simulink model "EST"  (R2025a)
settings: Solver=FixedStepAuto  StartTime=0.0  StopTime=stopt  FixedStep=deltat  MaxStep=0.05  RelTol=1e-3
InitFcn:
  | clear all;
  | close all;
  | clc;
  | 
  | % add the data and script directories
  | addpath('data','scripts');
  | 
  | % load the constants (units)
  | constants;
  | 
  | % load the simulation parameters
  | preprocessing;
StopFcn:
  | postprocessing;
values from neighbouring files (symbols this model uses):
  aDemandTransport = 0.01    [preprocessing.m]
  aInjection = 0.2    [preprocessing.m]
  aSupplyTransport = 0.01    [preprocessing.m]
  bStorage = (1/(ro*V*c*Rtb))/unit("s")    [preprocessing.m]
  EStorageInitial = 0.0*unit("MWh")    [preprocessing.m]
  EStorageMax = 107.*unit("MWh")    [preprocessing.m]
  EStorageMin = 0.1*unit("MWh")    [preprocessing.m]
settings Model: Creator=joche  LastModifiedBy=20253517
settings DataIOCC: SaveFormat=Array  SaveOutput=off  ReturnWorkspaceOutputs=off
settings OptimizationCC: ReuseModelBlockBuffer=off
settings ModelReferenceCC: EnableRefExpFcnMdlSchedulingChecks=on
settings RTWCC: GPUComputeCapability=3.5

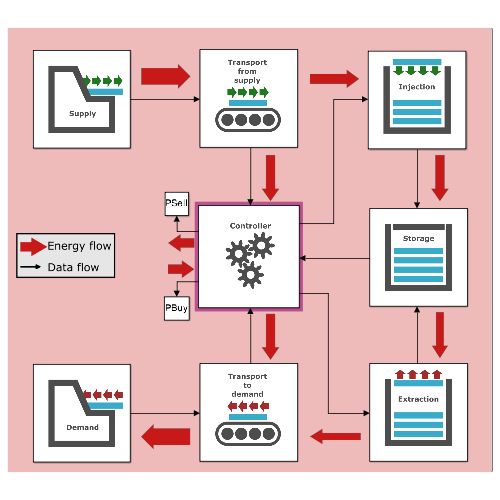
[thumbnail: Simulink's stored preview of the top-level diagram]
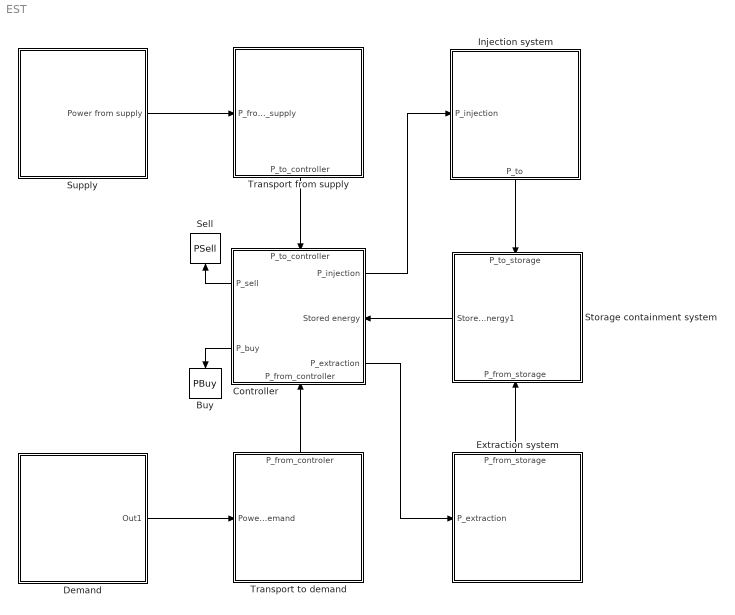
== system EST ==
  Buy : ToWorkspace  VariableName=PBuy  SampleTime=-1
  Controller : Subsystem
      settings: PortSchema="{\"entries\":[{\"content\":{\"sides\":[{\"content\":{\"connectorIds\":[\"Out3\",\"Out4\"]},\"type\":\"ConnectorPlacement.EquallySpacedRectSide\",\"uuid\":\"4daf33ce-c96a-4783-b5c4-228eed953e01\"},{\"content\":{\"connectorIds\":[\"Out1\",\"In3\",\"Out2\"],\"side\":\"RIGHT\"},\"type\":\"ConnectorPlacement.EquallySpacedRectSide\",\"uuid\":\"e9942e50-8467-4af8-b79b-80636cbc76e5\"},{\"content\":{\"connectorIds\":[\"In1\"],\"side\":\"TOP\"},\"type\":\"ConnectorPlacement.EquallySpacedRectSide\",\"uuid\":\"f315e931-d69b-4751-b712-f89c6c81baeb\"},{\"content\":{\"connectorIds\":[\"In2\"],\"side\":\"BOTTOM\"},\"type\":\"ConnectorPlacement.EquallySpacedRectSide\",\"uuid\":\"44715ee6-5cd5-4669-bcb9-5ed7c869bdb3\"}]},\"type\":\"ConnectorPlacement.EquallySpacedConnector\",\"uuid\":\"fff48899-944b-4064-b7d7-ecc12144fb48\"}],\"packageUris\":[\"http://schema.mathworks.com/mf0/Connector/R2020b\"],\"version\":\"1.0\"}"
      mask Display: image('$imagefile'); % Use "Edit Image" on toolstrip to change.
  Demand : Subsystem
      mask Display: image('$imagefile'); % Use "Edit Image" on toolstrip to change.
  Extraction system : Subsystem
      settings: PortSchema="{\"entries\":[{\"content\":{\"sides\":[{\"content\":{\"connectorIds\":[]},\"type\":\"ConnectorPlacement.EquallySpacedRectSide\",\"uuid\":\"05c5933d-55fc-4e06-853f-fc26d42905f9\"},{\"content\":{\"connectorIds\":[\"In1\"],\"side\":\"RIGHT\"},\"type\":\"ConnectorPlacement.EquallySpacedRectSide\",\"uuid\":\"327426c5-31d5-498b-a2bd-83e49353408c\"},{\"content\":{\"connectorIds\":[],\"side\":\"TOP\"},\"type\":\"ConnectorPlacement.EquallySpacedRectSide\",\"uuid\":\"55306cf3-a3de-4385-a5ae-b8600ecdd5a2\"},{\"content\":{\"connectorIds\":[\"Out1\"],\"side\":\"BOTTOM\"},\"type\":\"ConnectorPlacement.EquallySpacedRectSide\",\"uuid\":\"08fcc9c3-40d3-4ac6-b914-dfeef6039ffb\"}]},\"type\":\"ConnectorPlacement.EquallySpacedConnector\",\"uuid\":\"cb35d5ba-e8c6-462c-b7b2-fe8356d4b0a1\"}],\"packageUris\":[\"http://schema.mathworks.com/mf0/Connector/R2020b\"],\"version\":\"1.0\"}"
      mask Display: image('$imagefile'); % Use "Edit Image" on toolstrip to change.
  Injection system : Subsystem
      settings: PortSchema="{\"entries\":[{\"content\":{\"sides\":[{\"content\":{\"connectorIds\":[]},\"type\":\"ConnectorPlacement.EquallySpacedRectSide\",\"uuid\":\"05c5933d-55fc-4e06-853f-fc26d42905f9\"},{\"content\":{\"connectorIds\":[\"In1\"],\"side\":\"RIGHT\"},\"type\":\"ConnectorPlacement.EquallySpacedRectSide\",\"uuid\":\"327426c5-31d5-498b-a2bd-83e49353408c\"},{\"content\":{\"connectorIds\":[\"Out1\"],\"side\":\"TOP\"},\"type\":\"ConnectorPlacement.EquallySpacedRectSide\",\"uuid\":\"55306cf3-a3de-4385-a5ae-b8600ecdd5a2\"},{\"content\":{\"connectorIds\":[],\"side\":\"BOTTOM\"},\"type\":\"ConnectorPlacement.EquallySpacedRectSide\",\"uuid\":\"08fcc9c3-40d3-4ac6-b914-dfeef6039ffb\"}]},\"type\":\"ConnectorPlacement.EquallySpacedConnector\",\"uuid\":\"cb35d5ba-e8c6-462c-b7b2-fe8356d4b0a1\"}],\"packageUris\":[\"http://schema.mathworks.com/mf0/Connector/R2020b\"],\"version\":\"1.0\"}"
      mask Display: image('$imagefile'); % Use "Edit Image" on toolstrip to change.
  Sell : ToWorkspace  VariableName=PSell  SampleTime=-1
  Storage containment system : Subsystem
      settings: PortSchema="{\"entries\":[{\"content\":{\"sides\":[{\"content\":{\"connectorIds\":[\"Out1\"]},\"type\":\"ConnectorPlacement.EquallySpacedRectSide\",\"uuid\":\"0ba48424-33b9-4934-970f-64fe5d8b070e\"},{\"content\":{\"connectorIds\":[],\"side\":\"RIGHT\"},\"type\":\"ConnectorPlacement.EquallySpacedRectSide\",\"uuid\":\"9cde340f-8f39-4499-9a12-5e1623737660\"},{\"content\":{\"connectorIds\":[\"In1\"],\"side\":\"TOP\"},\"type\":\"ConnectorPlacement.EquallySpacedRectSide\",\"uuid\":\"2af8db04-7fd0-4902-8637-8dc00edb4598\"},{\"content\":{\"connectorIds\":[\"In2\"],\"side\":\"BOTTOM\"},\"type\":\"ConnectorPlacement.EquallySpacedRectSide\",\"uuid\":\"e21ea806-d777-41a3-a53f-556fae66854b\"}]},\"type\":\"ConnectorPlacement.EquallySpacedConnector\",\"uuid\":\"4e2ddb36-4db3-4ab4-858b-ebb8ccefeb1f\"}],\"packageUris\":[\"http://schema.mathworks.com/mf0/Connector/R2020b\"],\"version\":\"1.0\"}"
      mask Display: image('$imagefile'); % Use "Edit Image" on toolstrip to change.
  Supply : Subsystem
      mask Display: image('$imagefile'); % Use "Edit Image" on toolstrip to change.
  Transport from supply : Subsystem
      settings: PortSchema="{\"entries\":[{\"content\":{\"sides\":[{\"content\":{\"connectorIds\":[\"In1\"]},\"type\":\"ConnectorPlacement.EquallySpacedRectSide\",\"uuid\":\"31329006-3d36-4d93-9c44-7503a515d397\"},{\"content\":{\"connectorIds\":[],\"side\":\"RIGHT\"},\"type\":\"ConnectorPlacement.EquallySpacedRectSide\",\"uuid\":\"aba139c7-f9b6-4881-a56b-a4cbbedacd88\"},{\"content\":{\"connectorIds\":[],\"side\":\"TOP\"},\"type\":\"ConnectorPlacement.EquallySpacedRectSide\",\"uuid\":\"e683eb73-7a35-4160-9c39-da83856a6278\"},{\"content\":{\"connectorIds\":[\"Out1\"],\"side\":\"BOTTOM\"},\"type\":\"ConnectorPlacement.EquallySpacedRectSide\",\"uuid\":\"1170dd18-447c-437f-9043-6812c2877331\"}]},\"type\":\"ConnectorPlacement.EquallySpacedConnector\",\"uuid\":\"804af608-1d70-444f-af69-e05f19bf98f3\"}],\"packageUris\":[\"http://schema.mathworks.com/mf0/Connector/R2020b\"],\"version\":\"1.0\"}"
      mask Display: image('$imagefile'); % Use "Edit Image" on toolstrip to change.
  Transport to demand : Subsystem
      settings: PortSchema="{\"entries\":[{\"content\":{\"sides\":[{\"content\":{\"connectorIds\":[\"In1\"]},\"type\":\"ConnectorPlacement.EquallySpacedRectSide\",\"uuid\":\"31329006-3d36-4d93-9c44-7503a515d397\"},{\"content\":{\"connectorIds\":[],\"side\":\"RIGHT\"},\"type\":\"ConnectorPlacement.EquallySpacedRectSide\",\"uuid\":\"aba139c7-f9b6-4881-a56b-a4cbbedacd88\"},{\"content\":{\"connectorIds\":[\"Out1\"],\"side\":\"TOP\"},\"type\":\"ConnectorPlacement.EquallySpacedRectSide\",\"uuid\":\"e683eb73-7a35-4160-9c39-da83856a6278\"},{\"content\":{\"connectorIds\":[],\"side\":\"BOTTOM\"},\"type\":\"ConnectorPlacement.EquallySpacedRectSide\",\"uuid\":\"c378138f-7233-4483-870c-40a69b3495ee\"}]},\"type\":\"ConnectorPlacement.EquallySpacedConnector\",\"uuid\":\"804af608-1d70-444f-af69-e05f19bf98f3\"}],\"packageUris\":[\"http://schema.mathworks.com/mf0/Connector/R2020b\"],\"version\":\"1.0\"}"
      mask Display: image('$imagefile'); % Use "Edit Image" on toolstrip to change.
  wires:
  Supply/1(Power from supply) -> Transport from supply/1(P_from_supply)
  Transport from supply/1(P_to_controller) -> Controller/1(P_to_controller)
  Transport to demand/1(P_from_controler) -> Controller/2(P_from_controller)
  Demand/1(Out1) -> Transport to demand/1(Power to demand)
  Controller/3(P_sell) -> Sell/1
  Controller/2(P_extraction) -> Extraction system/1(P_extraction)
  Injection system/1(P_to) -> Storage containment system/1(P_to_storage)
  Extraction system/1(P_from_storage) -> Storage containment system/2(P_from_storage)
  Storage containment system/1(Stored energy1) -> Controller/3(Stored energy)
  Controller/1(P_injection) -> Injection system/1(P_injection)
  Controller/4(P_buy) -> Buy/1

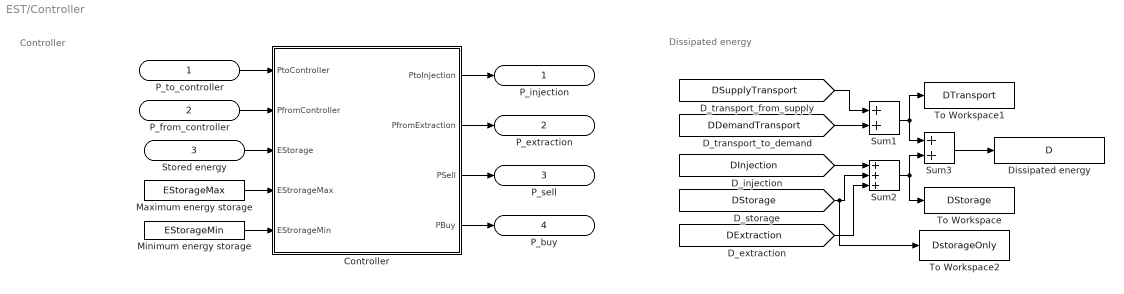
== system EST/Controller ==
  note: Dissipated energy
  note: Controller
  P_to_controller : Inport
  P_from_controller : Inport  Port=2
  Stored energy : Inport  Port=3
  Controller : MATLAB Function  TreatAsAtomicUnit=on
  Dissipated energy : ToWorkspace  VariableName=D  SampleTime=-1
  Maximum energy storage : Constant  Value=EStorageMax
  Minimum energy storage : Constant  Value=EStorageMin
  Sum1 : Sum
  Sum2 : Sum  Inputs=+++
  Sum3 : Sum
  To Workspace : ToWorkspace  VariableName=DStorage  SampleTime=-1
  To Workspace1 : ToWorkspace  VariableName=DTransport  SampleTime=-1
  To Workspace2 : ToWorkspace  VariableName=DstorageOnly  SampleTime=-1
  P_injection : Outport
  P_extraction : Outport  Port=2
  P_sell : Outport  Port=3
  P_buy : Outport  Port=4
  wires:
  P_from_controller/1 -> Controller/2(PfromController)
  Controller/2(PfromExtraction) -> P_extraction/1
  Controller/3(PSell) -> P_sell/1
  Controller/4(PBuy) -> P_buy/1
  Minimum energy storage/1 -> Controller/5(EStrorageMin)
  Maximum energy storage/1 -> Controller/4(EStrorageMax)
  P_to_controller/1 -> Controller/1(PtoController)
  Controller/1(PtoInjection) -> P_injection/1
  Stored energy/1 -> Controller/3(EStorage)
  [DDemandTransport] -> Sum1/2
  [DSupplyTransport] -> Sum1/1
  [DInjection] -> Sum2/1
  [DStorage] -> To Workspace2/1, Sum2/2
  [DExtraction] -> Sum2/3
  Sum2/1 -> To Workspace/1, Sum3/2
  Sum1/1 -> To Workspace1/1, Sum3/1
  Sum3/1 -> Dissipated energy/1

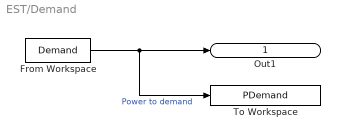
== system EST/Demand ==
  From Workspace : FromWorkspace  VariableName=Demand  OutputAfterFinalValue=Setting to zero
  To Workspace : ToWorkspace  VariableName=PDemand  SampleTime=-1
  Out1 : Outport
  wires:
  From Workspace/1 -> To Workspace/1, Out1/1  "Power to demand"

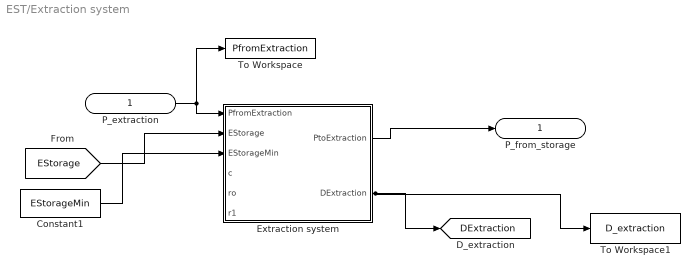
== system EST/Extraction system ==
  P_extraction : Inport
  Constant1 : Constant  Value=EStorageMin
  Extraction system : MATLAB Function  TreatAsAtomicUnit=on
  To Workspace : ToWorkspace  VariableName=PfromExtraction  SampleTime=-1
  To Workspace1 : ToWorkspace  VariableName=D_extraction  SampleTime=-1
  P_from_storage : Outport
  tag scope: DExtraction=global
  wires:
  P_extraction/1 -> To Workspace/1, Extraction system/1(PfromExtraction)
  Extraction system/1(PtoExtraction) -> P_from_storage/1
  [EStorage] -> Extraction system/2(EStorage)
  Constant1/1 -> Extraction system/3(EStorageMin)
  Extraction system/2(DExtraction) -> To Workspace1/1, [DExtraction]

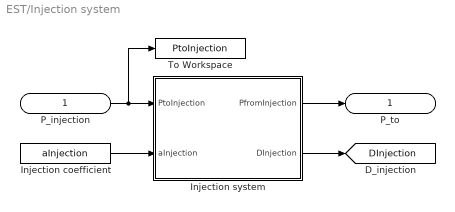
== system EST/Injection system ==
  P_injection : Inport
  Injection coefficient : Constant  Value=aInjection
  Injection system : MATLAB Function  TreatAsAtomicUnit=on
  To Workspace : ToWorkspace  VariableName=PtoInjection  SampleTime=-1
  P_to : Outport
  tag scope: DInjection=global
  wires:
  P_injection/1 -> To Workspace/1, Injection system/1(PtoInjection)
  Injection system/1(PfromInjection) -> P_to/1
  Injection coefficient/1 -> Injection system/2(aInjection)
  Injection system/2(DInjection) -> [DInjection]

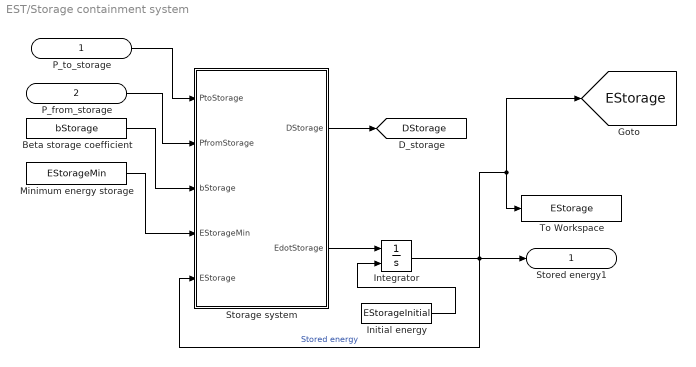
== system EST/Storage containment system ==
  P_to_storage : Inport
  P_from_storage : Inport  Port=2
  Beta storage coefficient : Constant  Value=bStorage
  Initial energy : Constant  Value=EStorageInitial
  Integrator : Integrator  InitialConditionSource=external
  Minimum energy storage : Constant  Value=EStorageMin
  Storage system : MATLAB Function  TreatAsAtomicUnit=on
  To Workspace : ToWorkspace  VariableName=EStorage  SampleTime=-1
  Stored energy1 : Outport
  tag scope: DStorage=global, EStorage=global
  wires:
  P_from_storage/1 -> Storage system/2(PfromStorage)
  P_to_storage/1 -> Storage system/1(PtoStorage)
  Initial energy/1 -> Integrator/2
  Integrator/1 -> [EStorage], To Workspace/1, Storage system/5(EStorage), Stored energy1/1  "Stored energy"
  Storage system/1(DStorage) -> [DStorage]
  Beta storage coefficient/1 -> Storage system/3(bStorage)
  Storage system/2(EdotStorage) -> Integrator/1
  Minimum energy storage/1 -> Storage system/4(EStorageMin)

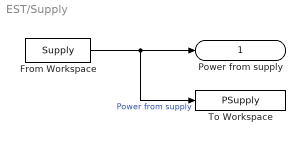
== system EST/Supply ==
  From Workspace : FromWorkspace  VariableName=Supply  OutputAfterFinalValue=Setting to zero
  To Workspace : ToWorkspace  VariableName=PSupply  SampleTime=-1
  Power from supply : Outport
  wires:
  From Workspace/1 -> To Workspace/1, Power from supply/1  "Power from supply"

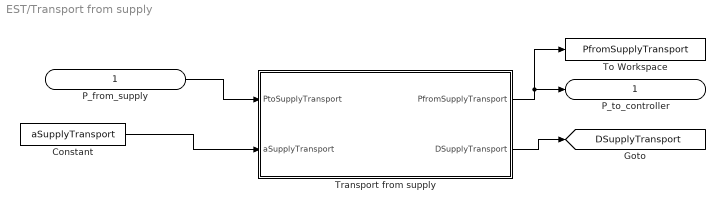
== system EST/Transport from supply ==
  P_from_supply : Inport
  Constant : Constant  Value=aSupplyTransport
  To Workspace : ToWorkspace  VariableName=PfromSupplyTransport  SampleTime=-1
  Transport from supply : MATLAB Function  TreatAsAtomicUnit=on
  P_to_controller : Outport
  tag scope: DSupplyTransport=global
  wires:
  P_from_supply/1 -> Transport from supply/1(PtoSupplyTransport)
  Transport from supply/1(PfromSupplyTransport) -> To Workspace/1, P_to_controller/1
  Transport from supply/2(DSupplyTransport) -> [DSupplyTransport]
  Constant/1 -> Transport from supply/2(aSupplyTransport)

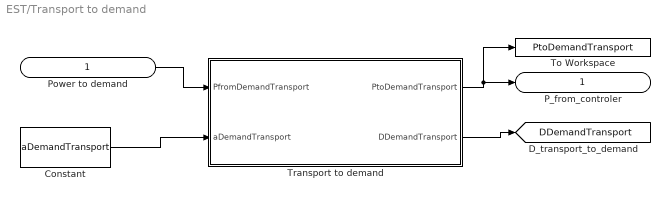
== system EST/Transport to demand ==
  Power to demand : Inport
  Constant : Constant  Value=aDemandTransport
  To Workspace : ToWorkspace  VariableName=PtoDemandTransport  SampleTime=-1
  Transport to demand : MATLAB Function  TreatAsAtomicUnit=on
  P_from_controler : Outport
  tag scope: DDemandTransport=global
  wires:
  Power to demand/1 -> Transport to demand/1(PfromDemandTransport)
  Transport to demand/1(PtoDemandTransport) -> To Workspace/1, P_from_controler/1
  Transport to demand/2(DDemandTransport) -> [DDemandTransport]
  Constant/1 -> Transport to demand/2(aDemandTransport)

== matlab function EST/Injection system/Injection system ==
  data: PtoInjection input; PfromInjection output; aInjection input; DInjection output
function [PfromInjection, DInjection] = injection(PtoInjection, aInjection)
    DInjection = aInjection * PtoInjection;
    PfromInjection = PtoInjection - DInjection;

== matlab function EST/Transport from supply/Transport from supply ==
  data: PtoSupplyTransport input; PfromSupplyTransport output; aSupplyTransport input; DSupplyTransport output
function [PfromSupplyTransport, DSupplyTransport] = supplyTransport(PtoSupplyTransport, aSupplyTransport)
    
    DSupplyTransport = aSupplyTransport* PtoSupplyTransport;
    PfromSupplyTransport = PtoSupplyTransport - DSupplyTransport;

== matlab function EST/Controller/Controller ==
  data: PtoInjection output; PfromExtraction output; PSell output; PBuy output; PtoController input; PfromController input; EStorage input; EStrorageMax input; EStrorageMin input
function [PtoInjection, PfromExtraction, PSell, PBuy] = controller(PtoController, PfromController, EStorage, EStrorageMax, EStrorageMin)
    
    %% Power surplus or deficit

    deltaP = PtoController - PfromController;

    % Power surplus
    if deltaP >= 0

        %% Storage injection

        % Storage system is not full
        if EStorage < EStrorageMax 

            PtoInjection = deltaP;

        % Storage system is full
        else
            PtoInjection = 0;
        end

        %% Storage extraction

        PfromExtraction = 0;

        %% Load-balancing
        PSell   = deltaP - PtoInjection;
        PBuy    = 0;

    % Power deficit
    else

        %% Storage injection

        PtoInjection = 0;

        %% Storage extraction

        % Storage system is not empty
        if EStorage > EStrorageMin

            PfromExtraction = -deltaP;

        % Storage system is empty
        else
            PfromExtraction = 0;
        end

        %% Load-balancing

        PSell = 0;
        PBuy  = -deltaP - PfromExtraction;
    end

== matlab function EST/Extraction system/Extraction system ==
  data: PfromExtraction input; PtoExtraction output; DExtraction output; EStorage input; EStorageMin input; c input; ro input; r1 input
function [PtoExtraction, DExtraction] = extraction(PfromExtraction, EStorage, EStorageMin,c , ro, r1)
    
     
    tHot = ((EStorage - EStorageMin)/(((4*pi/3)*c*ro*(r1^3))+285.15));
    
    eExtraction = 1 - 285.15/ tHot  ;

    DExtraction = eExtraction*PfromExtraction;

    PtoExtraction = PfromExtraction + DExtraction;

== matlab function EST/Storage containment system/Storage system ==
  data: DStorage output; EdotStorage output; PtoStorage input; PfromStorage input; bStorage input; EStorageMin input; EStorage input
function [DStorage, EdotStorage]= Storage(PtoStorage, PfromStorage, bStorage, EStorageMin, EStorage)


    DStorage = bStorage * (EStorage-EStorageMin);
    EdotStorage = PtoStorage - PfromStorage - DStorage;

== matlab function EST/Transport to demand/Transport to demand ==
  data: PfromDemandTransport input; PtoDemandTransport output; aDemandTransport input; DDemandTransport output
function [PtoDemandTransport, DDemandTransport] = demandTransport(PfromDemandTransport, aDemandTransport)
    
    DDemandTransport =  aDemandTransport*PfromDemandTransport;
    
    PtoDemandTransport = PfromDemandTransport + aDemandTransport;
